simulink model "time_law"  (R2024b)
settings: Solver=VariableStepAuto  StartTime=0.0  StopTime=10.0  RelTol=1e-3
settings Model: Creator=Riccardo  LastModifiedBy=Riccardo

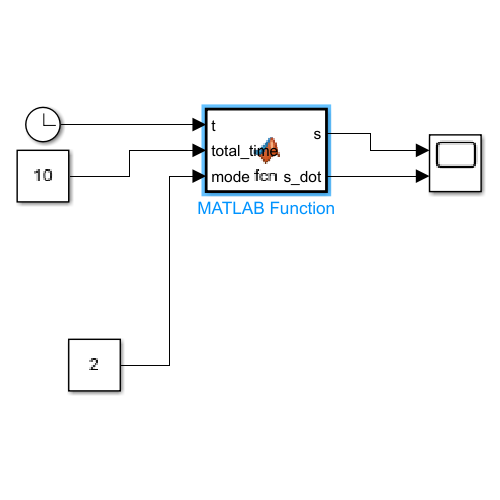
[thumbnail: Simulink's stored preview of the top-level diagram]
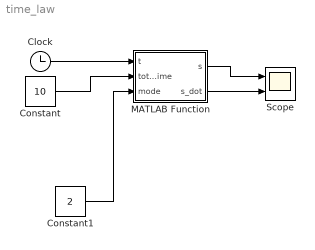
== system time_law ==
  Clock : Clock
      settings: Decimation=100
  Constant : Constant  Value=10
  Constant1 : Constant  Value=2
  MATLAB Function : MATLAB Function  TreatAsAtomicUnit=on
  Scope : Scope  NumInputPorts=2
  wires:
  Clock/1 -> MATLAB Function/1(t)
  Constant/1 -> MATLAB Function/2(total_time)
  Constant1/1 -> MATLAB Function/3(mode)
  MATLAB Function/1(s) -> Scope/1
  MATLAB Function/2(s_dot) -> Scope/2

== matlab function time_law/MATLAB Function ==
  data: t input; s output; total_time input; mode input; s_dot output
function [s, s_dot] = fcn(t,total_time,mode)
s=0;
s_dot=0;
if mode==1%if mode =1 costasnt time law else trapezoidal
    s_dot = 1/total_time;
    s=t/total_time;
else
    Ta=0.1*total_time;% acceleration/dec time 10% of total
    Tc=total_time-2*Ta;%time of costant time

    Vc=1/(Ta+Tc);% velocità costante
    a=Vc/Ta;% acceleration
    switch 1 %formula on the slide
        case t<Ta
            s_dot=a*t;
            s=(a*(t^2))/2;

        case (t>=Ta)&&(t<(Tc+Ta))
            s_dot=Vc;
            s=(a*(Ta^2))/2+Vc*(t-Ta);

        case (t>=(Tc+Ta))&&(t<(Tc+2*Ta))
            s_dot=Vc-a*(t-Ta-Tc);
            s=(a*(Ta^2))/2+Vc*Tc+Vc*(t-Ta-Tc)-a*(t-Ta-Tc)^2/2;

        case t>=(Tc+2*Ta)
            s_dot=0;
            s=1;
    end

end
